simulink subsystem "innerLoop"  (R2026a)
settings: Solver=VariableStepAuto
settings Model: Creator=maxhu  LastModifiedBy=maxhu

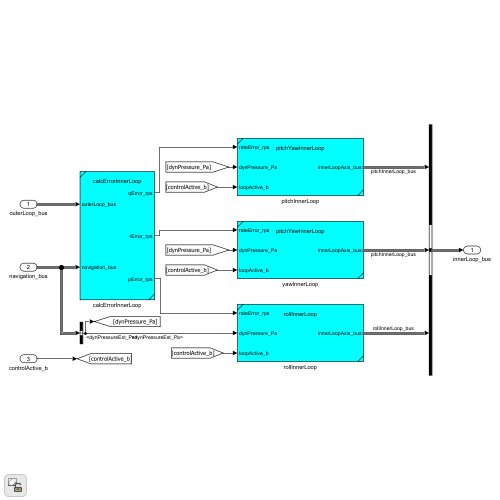
[thumbnail: Simulink's stored preview of the top-level diagram]
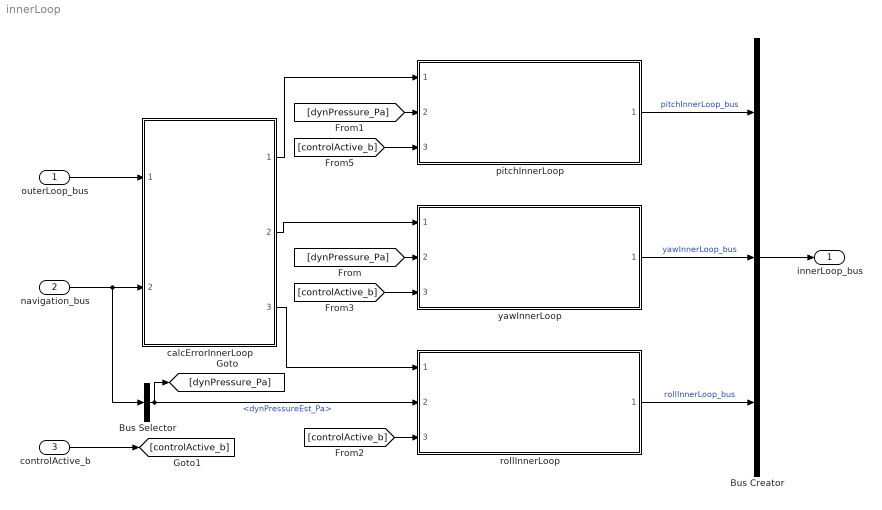
== system innerLoop ==
  outerLoop_bus : Inport
  navigation_bus : Inport  Port=2
  controlActive_b : Inport  Port=3
  Bus Creator : BusCreator  Inputs=3
  Bus Selector : BusSelector  OutputSignals=dynPressureEst_Pa
  calcErrorInnerLoop : Subsystem  ReferencedSubsystem=calcErrorInnerLoop
  pitchInnerLoop : Subsystem  ReferencedSubsystem=pitchYawInnerLoop
      settings: PermitHierarchicalResolution=None
  rollInnerLoop : Subsystem  ReferencedSubsystem=rollInnerLoop
      settings: PermitHierarchicalResolution=None
  yawInnerLoop : Subsystem  ReferencedSubsystem=pitchYawInnerLoop
      settings: PermitHierarchicalResolution=None
  innerLoop_bus : Outport
  wires:
  [dynPressure_Pa] -> pitchInnerLoop/2
  rollInnerLoop/1 -> Bus Creator/3  "rollInnerLoop_bus"
  pitchInnerLoop/1 -> Bus Creator/1  "pitchInnerLoop_bus"
  calcErrorInnerLoop/3 -> rollInnerLoop/1
  Bus Creator/1 -> innerLoop_bus/1
  outerLoop_bus/1 -> calcErrorInnerLoop/1
  navigation_bus/1 -> calcErrorInnerLoop/2, Bus Selector/1
  Bus Selector/1 -> [dynPressure_Pa], rollInnerLoop/2  "<dynPressureEst_Pa>"
  calcErrorInnerLoop/1 -> pitchInnerLoop/1
  controlActive_b/1 -> [controlActive_b]
  [controlActive_b] -> rollInnerLoop/3
  [controlActive_b] -> pitchInnerLoop/3
  [dynPressure_Pa] -> yawInnerLoop/2
  calcErrorInnerLoop/2 -> yawInnerLoop/1
  [controlActive_b] -> yawInnerLoop/3
  yawInnerLoop/1 -> Bus Creator/2  "yawInnerLoop_bus"
